simulink model "tppr2"  (R2020a)
settings: Solver=ode45  StartTime=0.0  StopTime=10  RelTol=1e-8
libraries: simulink x4
settings Model: Creator=dot  LastModifiedBy=dot

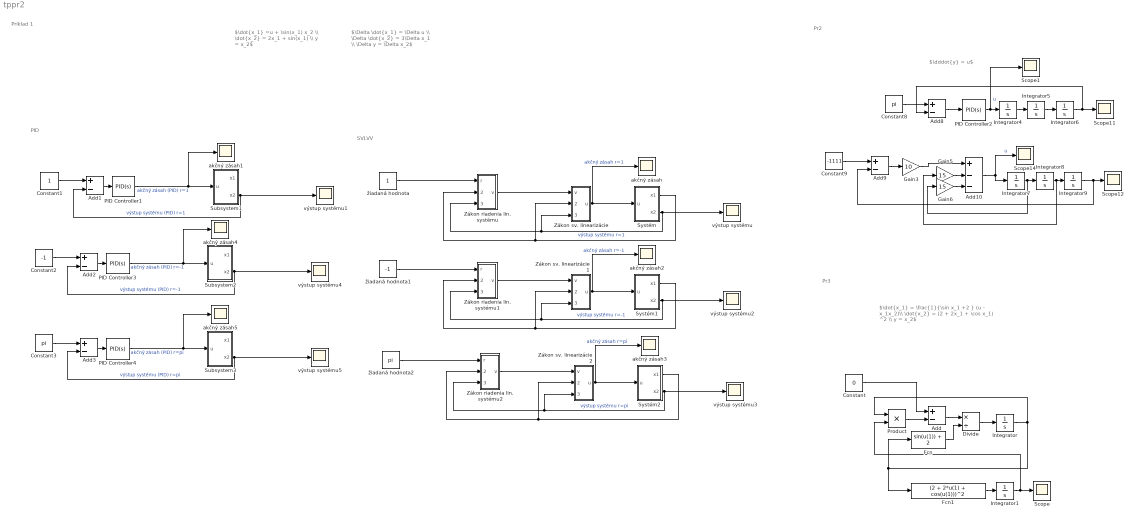
== system tppr2 ==
  note: Pr3
  note: Pr2
  note: Príklad 1
  note: SVLVV
  note: PID
  note: $\dot{x_1} =u + \sin(x_1) x_2 \\ \dot{x_2} = 2x_1 + sin(x_1) \\ y = x_2$
  note: $\dddot{y} = u$
  note: $\dot{x_1} = \frac{1}{\sin x_1 +2 } (u - x_1x_2)\\ \dot{x_2} = (2 + 2x_1 + \cos x_1) ^2 \\ y = x_2$
  note: $\Delta \dot{x_1} = \Delta u \\ \Delta \dot{x_2} = 3\Delta x_1 \\ \Delta y = \Delta x_2$
  Add{,1..3,8..9} (6 alike) : Sum  Inputs=+-
  Add10 : Sum  Inputs=+--
  Constant : Constant  Value=0
  Constant1 : Constant
  Constant2 : Constant  Value=-1
  Constant3 : Constant  Value=pi
  Constant8 : Constant  Value=pi
  Constant9 : Constant  Value=-1111
  Divide : Product  Inputs=*/
  Fcn : Fcn  Expr=sin(u(1)) + 2
  Fcn1 : Fcn  Expr=(2 + 2*u(1) + cos(u(1)))^2
  Gain3 : Gain  Gain=10
  Gain5 : Gain  Gain=15
  Gain6 : Gain  Gain=15
  Integrator : Integrator  InitialCondition=-1.18715
  Integrator1 : Integrator
  Integrator{4..9} (6 alike) : Integrator  InitialCondition=pi/2
  PID Controller1 : simulink/Continuous/PID Controller  Controller=PID  Form=Parallel  TimeDomain=Continuous-time  UseExternalTs=off  SampleTime=-1  IntegratorMethod=Forward Euler  FilterMethod=Forward Euler  ControllerParametersSource=internal  P=2/3  I=1.25/3  D=0.25/3  UseFilter=on  N=114.28279760416  TunerSelectOption=Transfer Function Based (PID Tuner App)  InitialConditionSource=internal  InitialConditionForIntegrator=0  InitialConditionForFilter=0  DifferentiatorICPrevScaledInput=0  ExternalReset=none  TrackingMode=off  Kt=1  LimitOutput=off  UpperSaturationLimit=inf  LowerSaturationLimit=-inf  LinearizeAsGain=on  AntiWindupMode=none  Kb=1  POutMin=[]  POutMax=[]  IOutMin=[]  IOutMax=[]  DOutMin=[]  DOutMax=[]  NOutMin=[]  NOutMax=[]  SumOutMin=[]  SumOutMax=[]  SaturationOutMin=[]  SaturationOutMax=[]  PParamMin=[]  PParamMax=[]  IParamMin=[]  IParamMax=[]  DParamMin=[]  DParamMax=[]  NParamMin=[]  NParamMax=[]  KbParamMin=[]  KbParamMax=[]  KtParamMin=[]  KtParamMax=[]  KbOutMin=[]  KbOutMax=[]  KtOutMin=[]  KtOutMax=[]  IntegratorOutMin=[]  IntegratorOutMax=[]  FilterOutMin=[]  FilterOutMax=[]  SumI1OutMin=[]  SumI1OutMax=[]  SumI2OutMin=[]  SumI2OutMax=[]  SumI3OutMin=[]  SumI3OutMax=[]  SumI4OutMin=[]  SumI4OutMax=[]  SumDOutMin=[]  SumDOutMax=[]  DifferentiatorOutMin=[]  DifferentiatorOutMax=[]  FilterDiffOutCoefMin=[]  FilterDiffOutCoefMax=[]  ReciprocalOutMin=[]  ReciprocalOutMax=[]  SumDenOutMin=[]  SumDenOutMax=[]  SumNumOutMin=[]  SumNumOutMax=[]  DivideOutMin=[]  DivideOutMax=[]  UdiffTsProdOutMin=[]  UdiffTsProdOutMax=[]  NTsProdOutMin=[]  NTsProdOutMax=[]  UintegralTsProdOutMin=[]  UintegralTsProdOutMax=[]  UngainTsProdOutMin=[]  UngainTsProdOutMax=[]  IntegratorContinuousStateAttributes=''  IntegratorStateMustResolveToSignalObject=off  IntegratorRTWStateStorageClass=Auto  FilterContinuousStateAttributes=''  FilterStateMustResolveToSignalObject=off  FilterRTWStateStorageClass=Auto  ParallelPVariant=InternalParameters  IdealPVariant=Disabled  IVariant=InternalParameters  DVariant=InternalParameters  IntegratorVariant=Continuous  SatVariant=Disabled  AWVariant=Passthrough  PCopyVariant=Disabled  TRVariant=Disabled  FdbkBlocksVariant=Forward  IdealPFdbkVariant=Disabled  SatFdbkVariant=Disabled  DerivativeFilterVariant=ContFilter  NVariant=InternalParameters  NCopyVariant=Disabled  FilterICVariant=InternalICsFilter  IntegratorICVariant=InternalICs  ExternalResetVariant=Disabled  TRSumVariant=Passthrough  SumFdbkVariant=Disabled  SumVariant=Sum_PID  TsampFilterVariant=InternalTs  TsampNgainVariant=Passthrough  TsampIntegralVariant=Passthrough
  PID Controller2 : simulink/Continuous/PID Controller  Controller=PID  Form=Parallel  TimeDomain=Continuous-time  UseExternalTs=off  SampleTime=-1  IntegratorMethod=Forward Euler  FilterMethod=Forward Euler  ControllerParametersSource=internal  P=20.1650988848254  I=19.5294021366559  D=3.60985208452342  UseFilter=on  N=386.119892426795  TunerSelectOption=Transfer Function Based (PID Tuner App)  InitialConditionSource=internal  InitialConditionForIntegrator=0  InitialConditionForFilter=0  DifferentiatorICPrevScaledInput=0  ExternalReset=none  TrackingMode=off  Kt=1  LimitOutput=off  UpperSaturationLimit=inf  LowerSaturationLimit=-inf  LinearizeAsGain=on  AntiWindupMode=none  Kb=1  POutMin=[]  POutMax=[]  IOutMin=[]  IOutMax=[]  DOutMin=[]  DOutMax=[]  NOutMin=[]  NOutMax=[]  SumOutMin=[]  SumOutMax=[]  SaturationOutMin=[]  SaturationOutMax=[]  PParamMin=[]  PParamMax=[]  IParamMin=[]  IParamMax=[]  DParamMin=[]  DParamMax=[]  NParamMin=[]  NParamMax=[]  KbParamMin=[]  KbParamMax=[]  KtParamMin=[]  KtParamMax=[]  KbOutMin=[]  KbOutMax=[]  KtOutMin=[]  KtOutMax=[]  IntegratorOutMin=[]  IntegratorOutMax=[]  FilterOutMin=[]  FilterOutMax=[]  SumI1OutMin=[]  SumI1OutMax=[]  SumI2OutMin=[]  SumI2OutMax=[]  SumI3OutMin=[]  SumI3OutMax=[]  SumI4OutMin=[]  SumI4OutMax=[]  SumDOutMin=[]  SumDOutMax=[]  DifferentiatorOutMin=[]  DifferentiatorOutMax=[]  FilterDiffOutCoefMin=[]  FilterDiffOutCoefMax=[]  ReciprocalOutMin=[]  ReciprocalOutMax=[]  SumDenOutMin=[]  SumDenOutMax=[]  SumNumOutMin=[]  SumNumOutMax=[]  DivideOutMin=[]  DivideOutMax=[]  UdiffTsProdOutMin=[]  UdiffTsProdOutMax=[]  NTsProdOutMin=[]  NTsProdOutMax=[]  UintegralTsProdOutMin=[]  UintegralTsProdOutMax=[]  UngainTsProdOutMin=[]  UngainTsProdOutMax=[]  IntegratorContinuousStateAttributes=''  IntegratorStateMustResolveToSignalObject=off  IntegratorRTWStateStorageClass=Auto  FilterContinuousStateAttributes=''  FilterStateMustResolveToSignalObject=off  FilterRTWStateStorageClass=Auto  ParallelPVariant=InternalParameters  IdealPVariant=Disabled  IVariant=InternalParameters  DVariant=InternalParameters  IntegratorVariant=Continuous  SatVariant=Disabled  AWVariant=Passthrough  PCopyVariant=Disabled  TRVariant=Disabled  FdbkBlocksVariant=Forward  IdealPFdbkVariant=Disabled  SatFdbkVariant=Disabled  DerivativeFilterVariant=ContFilter  NVariant=InternalParameters  NCopyVariant=Disabled  FilterICVariant=InternalICsFilter  IntegratorICVariant=InternalICs  ExternalResetVariant=Disabled  TRSumVariant=Passthrough  SumFdbkVariant=Disabled  SumVariant=Sum_PID  TsampFilterVariant=InternalTs  TsampNgainVariant=Passthrough  TsampIntegralVariant=Passthrough
  PID Controller3 : simulink/Continuous/PID Controller  Controller=PID  Form=Parallel  TimeDomain=Continuous-time  UseExternalTs=off  SampleTime=-1  IntegratorMethod=Forward Euler  FilterMethod=Forward Euler  ControllerParametersSource=internal  P=2/3  I=1.25/3  D=0.25/3  UseFilter=on  N=114.28279760416  TunerSelectOption=Transfer Function Based (PID Tuner App)  InitialConditionSource=internal  InitialConditionForIntegrator=0  InitialConditionForFilter=0  DifferentiatorICPrevScaledInput=0  ExternalReset=none  TrackingMode=off  Kt=1  LimitOutput=off  UpperSaturationLimit=inf  LowerSaturationLimit=-inf  LinearizeAsGain=on  AntiWindupMode=none  Kb=1  POutMin=[]  POutMax=[]  IOutMin=[]  IOutMax=[]  DOutMin=[]  DOutMax=[]  NOutMin=[]  NOutMax=[]  SumOutMin=[]  SumOutMax=[]  SaturationOutMin=[]  SaturationOutMax=[]  PParamMin=[]  PParamMax=[]  IParamMin=[]  IParamMax=[]  DParamMin=[]  DParamMax=[]  NParamMin=[]  NParamMax=[]  KbParamMin=[]  KbParamMax=[]  KtParamMin=[]  KtParamMax=[]  KbOutMin=[]  KbOutMax=[]  KtOutMin=[]  KtOutMax=[]  IntegratorOutMin=[]  IntegratorOutMax=[]  FilterOutMin=[]  FilterOutMax=[]  SumI1OutMin=[]  SumI1OutMax=[]  SumI2OutMin=[]  SumI2OutMax=[]  SumI3OutMin=[]  SumI3OutMax=[]  SumI4OutMin=[]  SumI4OutMax=[]  SumDOutMin=[]  SumDOutMax=[]  DifferentiatorOutMin=[]  DifferentiatorOutMax=[]  FilterDiffOutCoefMin=[]  FilterDiffOutCoefMax=[]  ReciprocalOutMin=[]  ReciprocalOutMax=[]  SumDenOutMin=[]  SumDenOutMax=[]  SumNumOutMin=[]  SumNumOutMax=[]  DivideOutMin=[]  DivideOutMax=[]  UdiffTsProdOutMin=[]  UdiffTsProdOutMax=[]  NTsProdOutMin=[]  NTsProdOutMax=[]  UintegralTsProdOutMin=[]  UintegralTsProdOutMax=[]  UngainTsProdOutMin=[]  UngainTsProdOutMax=[]  IntegratorContinuousStateAttributes=''  IntegratorStateMustResolveToSignalObject=off  IntegratorRTWStateStorageClass=Auto  FilterContinuousStateAttributes=''  FilterStateMustResolveToSignalObject=off  FilterRTWStateStorageClass=Auto  ParallelPVariant=InternalParameters  IdealPVariant=Disabled  IVariant=InternalParameters  DVariant=InternalParameters  IntegratorVariant=Continuous  SatVariant=Disabled  AWVariant=Passthrough  PCopyVariant=Disabled  TRVariant=Disabled  FdbkBlocksVariant=Forward  IdealPFdbkVariant=Disabled  SatFdbkVariant=Disabled  DerivativeFilterVariant=ContFilter  NVariant=InternalParameters  NCopyVariant=Disabled  FilterICVariant=InternalICsFilter  IntegratorICVariant=InternalICs  ExternalResetVariant=Disabled  TRSumVariant=Passthrough  SumFdbkVariant=Disabled  SumVariant=Sum_PID  TsampFilterVariant=InternalTs  TsampNgainVariant=Passthrough  TsampIntegralVariant=Passthrough
  PID Controller4 : simulink/Continuous/PID Controller  Controller=PID  Form=Parallel  TimeDomain=Continuous-time  UseExternalTs=off  SampleTime=-1  IntegratorMethod=Forward Euler  FilterMethod=Forward Euler  ControllerParametersSource=internal  P=2/3  I=1.25/3  D=0.25/3  UseFilter=on  N=114.28279760416  TunerSelectOption=Transfer Function Based (PID Tuner App)  InitialConditionSource=internal  InitialConditionForIntegrator=0  InitialConditionForFilter=0  DifferentiatorICPrevScaledInput=0  ExternalReset=none  TrackingMode=off  Kt=1  LimitOutput=off  UpperSaturationLimit=inf  LowerSaturationLimit=-inf  LinearizeAsGain=on  AntiWindupMode=none  Kb=1  POutMin=[]  POutMax=[]  IOutMin=[]  IOutMax=[]  DOutMin=[]  DOutMax=[]  NOutMin=[]  NOutMax=[]  SumOutMin=[]  SumOutMax=[]  SaturationOutMin=[]  SaturationOutMax=[]  PParamMin=[]  PParamMax=[]  IParamMin=[]  IParamMax=[]  DParamMin=[]  DParamMax=[]  NParamMin=[]  NParamMax=[]  KbParamMin=[]  KbParamMax=[]  KtParamMin=[]  KtParamMax=[]  KbOutMin=[]  KbOutMax=[]  KtOutMin=[]  KtOutMax=[]  IntegratorOutMin=[]  IntegratorOutMax=[]  FilterOutMin=[]  FilterOutMax=[]  SumI1OutMin=[]  SumI1OutMax=[]  SumI2OutMin=[]  SumI2OutMax=[]  SumI3OutMin=[]  SumI3OutMax=[]  SumI4OutMin=[]  SumI4OutMax=[]  SumDOutMin=[]  SumDOutMax=[]  DifferentiatorOutMin=[]  DifferentiatorOutMax=[]  FilterDiffOutCoefMin=[]  FilterDiffOutCoefMax=[]  ReciprocalOutMin=[]  ReciprocalOutMax=[]  SumDenOutMin=[]  SumDenOutMax=[]  SumNumOutMin=[]  SumNumOutMax=[]  DivideOutMin=[]  DivideOutMax=[]  UdiffTsProdOutMin=[]  UdiffTsProdOutMax=[]  NTsProdOutMin=[]  NTsProdOutMax=[]  UintegralTsProdOutMin=[]  UintegralTsProdOutMax=[]  UngainTsProdOutMin=[]  UngainTsProdOutMax=[]  IntegratorContinuousStateAttributes=''  IntegratorStateMustResolveToSignalObject=off  IntegratorRTWStateStorageClass=Auto  FilterContinuousStateAttributes=''  FilterStateMustResolveToSignalObject=off  FilterRTWStateStorageClass=Auto  ParallelPVariant=InternalParameters  IdealPVariant=Disabled  IVariant=InternalParameters  DVariant=InternalParameters  IntegratorVariant=Continuous  SatVariant=Disabled  AWVariant=Passthrough  PCopyVariant=Disabled  TRVariant=Disabled  FdbkBlocksVariant=Forward  IdealPFdbkVariant=Disabled  SatFdbkVariant=Disabled  DerivativeFilterVariant=ContFilter  NVariant=InternalParameters  NCopyVariant=Disabled  FilterICVariant=InternalICsFilter  IntegratorICVariant=InternalICs  ExternalResetVariant=Disabled  TRSumVariant=Passthrough  SumFdbkVariant=Disabled  SumVariant=Sum_PID  TsampFilterVariant=InternalTs  TsampNgainVariant=Passthrough  TsampIntegralVariant=Passthrough
  Product : Product
  Scope{,1,11..12,14} (5 alike) : Scope
  Subsystem1 : Subsystem
  Subsystem2 : Subsystem
  Subsystem3 : Subsystem
  Systém : Subsystem
  Systém1 : Subsystem
  Systém2 : Subsystem
  Zákon riadenia lin. systému : Subsystem
  Zákon riadenia lin. systému1 : Subsystem
  Zákon riadenia lin. systému2 : Subsystem
  Zákon sv. linearizácie : Subsystem
  Zákon sv. linearizácie1 : Subsystem
  Zákon sv. linearizácie2 : Subsystem
  akčný zásah{,1..5} (6 alike) : Scope
  výstup systému{,1..5} (6 alike) : Scope
  žiadaná hodnota : Constant
  žiadaná hodnota1 : Constant  Value=-1
  žiadaná hodnota2 : Constant  Value=pi
  wires:
  Integrator4/1 -> Integrator5/1
  Integrator5/1 -> Integrator6/1
  Constant8/1 -> Add8/1
  Integrator6/1 -> Add8/2, Scope11/1
  Add8/1 -> PID Controller2/1
  PID Controller2/1 -> Scope1/1, Integrator4/1  "u"
  Add10/1 -> Scope14/1, Integrator7/1  "u"
  Integrator9/1 -> Scope12/1, Add9/2
  Constant9/1 -> Add9/1
  Integrator8/1 -> Gain5/1, Integrator9/1
  Integrator7/1 -> Gain6/1, Integrator8/1
  Add9/1 -> Gain3/1
  Gain3/1 -> Add10/1
  Gain5/1 -> Add10/2
  Gain6/1 -> Add10/3
  Zákon sv. linearizácie/1(u) -> akčný zásah/1, Systém/1(u)  "akčný zásah r=1"
  Systém/1(x1) -> Zákon sv. linearizácie/2(x1), Zákon riadenia lin. systému/2(x1)
  Systém/2(x2) -> výstup systému/1, Zákon sv. linearizácie/3(x2), Zákon riadenia lin. systému/3(x2)  "výstup systému r=1"
  Zákon riadenia lin. systému/1(v) -> Zákon sv. linearizácie/1(v)
  žiadaná hodnota/1 -> Zákon riadenia lin. systému/1(r)
  Product/1 -> Add/2
  Add/1 -> Divide/1
  Divide/1 -> Integrator/1
  Integrator/1 -> Fcn1/1, Fcn/1, Product/1
  Constant/1 -> Add/1
  Fcn/1 -> Divide/2
  Integrator1/1 -> Scope/1, Product/2
  Fcn1/1 -> Integrator1/1
  Constant1/1 -> Add1/1
  PID Controller1/1 -> Subsystem1/1(u), akčný zásah1/1  "akčný zásah (PID) r=1"
  Subsystem1/2(x2) -> výstup systému1/1, Add1/2  "výstup systému (PID) r=1"
  Add1/1 -> PID Controller1/1
  žiadaná hodnota1/1 -> Zákon riadenia lin. systému1/1(r)
  Zákon riadenia lin. systému1/1(v) -> Zákon sv. linearizácie1/1(v)
  Systém1/2(x2) -> Zákon riadenia lin. systému1/3(x2), Zákon sv. linearizácie1/3(x2), výstup systému2/1  "výstup systému r=-1"
  Systém1/1(x1) -> Zákon riadenia lin. systému1/2(x1), Zákon sv. linearizácie1/2(x1)
  Zákon sv. linearizácie1/1(u) -> Systém1/1(u), akčný zásah2/1  "akčný zásah r=-1"
  Zákon sv. linearizácie2/1(u) -> akčný zásah3/1, Systém2/1(u)  "akčný zásah r=pi"
  Systém2/1(x1) -> Zákon sv. linearizácie2/2(x1), Zákon riadenia lin. systému2/2(x1)
  Systém2/2(x2) -> výstup systému3/1, Zákon sv. linearizácie2/3(x2), Zákon riadenia lin. systému2/3(x2)  "výstup systému r=pi"
  Zákon riadenia lin. systému2/1(v) -> Zákon sv. linearizácie2/1(v)
  žiadaná hodnota2/1 -> Zákon riadenia lin. systému2/1(r)
  Add2/1 -> PID Controller3/1
  Subsystem2/2(x2) -> Add2/2, výstup systému4/1  "výstup systému (PID) r=-1"
  PID Controller3/1 -> akčný zásah4/1, Subsystem2/1(u)  "akčný zásah (PID) r=-1"
  Constant2/1 -> Add2/1
  Constant3/1 -> Add3/1
  PID Controller4/1 -> Subsystem3/1(u), akčný zásah5/1  "akčný zásah (PID) r=pi"
  Subsystem3/2(x2) -> výstup systému5/1, Add3/2  "výstup systému (PID) r=pi"
  Add3/1 -> PID Controller4/1

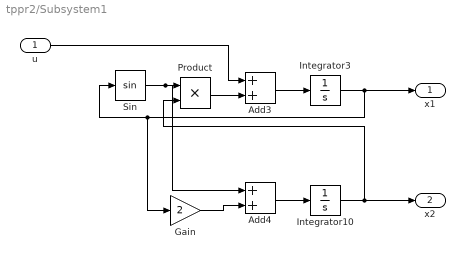
== system tppr2/Subsystem1 ==
  u : Inport
  Add3 : Sum
  Add4 : Sum
  Gain : Gain  Gain=2
  Integrator10 : Integrator
  Integrator3 : Integrator
  Product : Product
  Sin : Trigonometry
  x1 : Outport
  x2 : Outport  Port=2
  wires:
  Add4/1 -> Integrator10/1
  Gain/1 -> Add4/2
  u/1 -> Add3/1
  Add3/1 -> Integrator3/1
  Integrator3/1 -> Gain/1, Sin/1, x1/1
  Product/1 -> Add3/2
  Integrator10/1 -> Product/2, x2/1
  Sin/1 -> Add4/1, Product/1

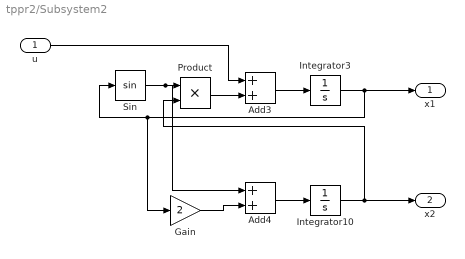
== system tppr2/Subsystem2 ==
  u : Inport
  Add3 : Sum
  Add4 : Sum
  Gain : Gain  Gain=2
  Integrator10 : Integrator
  Integrator3 : Integrator
  Product : Product
  Sin : Trigonometry
  x1 : Outport
  x2 : Outport  Port=2
  wires:
  Sin/1 -> Product/1, Add4/1
  Integrator10/1 -> x2/1, Product/2
  Product/1 -> Add3/2
  Integrator3/1 -> x1/1, Sin/1, Gain/1
  Add3/1 -> Integrator3/1
  u/1 -> Add3/1
  Gain/1 -> Add4/2
  Add4/1 -> Integrator10/1

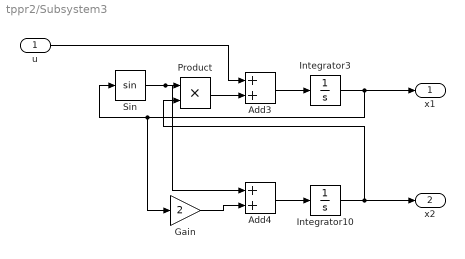
== system tppr2/Subsystem3 ==
  u : Inport
  Add3 : Sum
  Add4 : Sum
  Gain : Gain  Gain=2
  Integrator10 : Integrator
  Integrator3 : Integrator
  Product : Product
  Sin : Trigonometry
  x1 : Outport
  x2 : Outport  Port=2
  wires:
  Add4/1 -> Integrator10/1
  Gain/1 -> Add4/2
  u/1 -> Add3/1
  Add3/1 -> Integrator3/1
  Integrator3/1 -> Gain/1, Sin/1, x1/1
  Product/1 -> Add3/2
  Integrator10/1 -> Product/2, x2/1
  Sin/1 -> Add4/1, Product/1

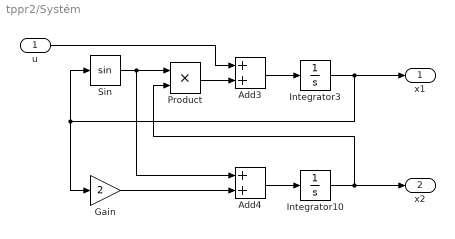
== system tppr2/Systém ==
  u : Inport
  Add3 : Sum
  Add4 : Sum
  Gain : Gain  Gain=2
  Integrator10 : Integrator
  Integrator3 : Integrator
  Product : Product
  Sin : Trigonometry
  x1 : Outport
  x2 : Outport  Port=2
  wires:
  Add4/1 -> Integrator10/1
  Gain/1 -> Add4/2
  u/1 -> Add3/1
  Add3/1 -> Integrator3/1
  Integrator3/1 -> Sin/1, Gain/1, x1/1
  Product/1 -> Add3/2
  Integrator10/1 -> Product/2, x2/1
  Sin/1 -> Product/1, Add4/1

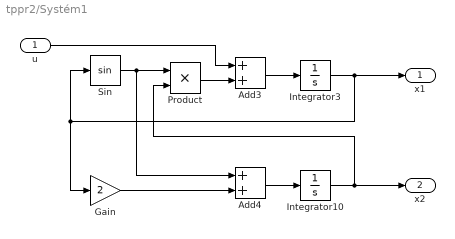
== system tppr2/Systém1 ==
  u : Inport
  Add3 : Sum
  Add4 : Sum
  Gain : Gain  Gain=2
  Integrator10 : Integrator
  Integrator3 : Integrator
  Product : Product
  Sin : Trigonometry
  x1 : Outport
  x2 : Outport  Port=2
  wires:
  Sin/1 -> Add4/1, Product/1
  Integrator10/1 -> x2/1, Product/2
  Product/1 -> Add3/2
  Integrator3/1 -> x1/1, Gain/1, Sin/1
  Add3/1 -> Integrator3/1
  u/1 -> Add3/1
  Gain/1 -> Add4/2
  Add4/1 -> Integrator10/1

== system tppr2/Systém2 ==
  u : Inport
  Add3 : Sum
  Add4 : Sum
  Gain : Gain  Gain=2
  Integrator10 : Integrator
  Integrator3 : Integrator
  Product : Product
  Sin : Trigonometry
  x1 : Outport
  x2 : Outport  Port=2
  wires:
  Add4/1 -> Integrator10/1
  Gain/1 -> Add4/2
  u/1 -> Add3/1
  Add3/1 -> Integrator3/1
  Integrator3/1 -> Sin/1, Gain/1, x1/1
  Product/1 -> Add3/2
  Integrator10/1 -> Product/2, x2/1
  Sin/1 -> Product/1, Add4/1

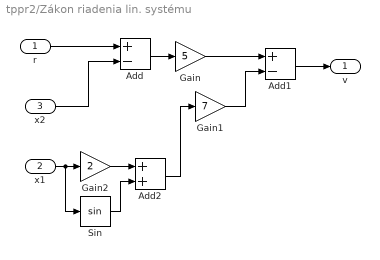
== system tppr2/Zákon riadenia lin. systému ==
  r : Inport
  x1 : Inport  Port=2
  x2 : Inport  Port=3
  Add : Sum  Inputs=+-
  Add1 : Sum  Inputs=+-
  Add2 : Sum
  Gain : Gain  Gain=5
  Gain1 : Gain  Gain=7
  Gain2 : Gain  Gain=2
  Sin : Trigonometry
  v : Outport
  wires:
  r/1 -> Add/1
  x1/1 -> Sin/1, Gain2/1
  Add/1 -> Gain/1
  Gain/1 -> Add1/1
  Add1/1 -> v/1
  Gain1/1 -> Add1/2
  Gain2/1 -> Add2/1
  Sin/1 -> Add2/2
  Add2/1 -> Gain1/1
  x2/1 -> Add/2

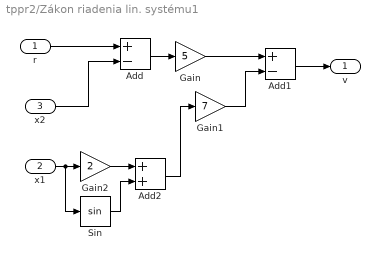
== system tppr2/Zákon riadenia lin. systému1 ==
  r : Inport
  x1 : Inport  Port=2
  x2 : Inport  Port=3
  Add : Sum  Inputs=+-
  Add1 : Sum  Inputs=+-
  Add2 : Sum
  Gain : Gain  Gain=5
  Gain1 : Gain  Gain=7
  Gain2 : Gain  Gain=2
  Sin : Trigonometry
  v : Outport
  wires:
  x2/1 -> Add/2
  Add2/1 -> Gain1/1
  Sin/1 -> Add2/2
  Gain2/1 -> Add2/1
  Gain1/1 -> Add1/2
  Add1/1 -> v/1
  Gain/1 -> Add1/1
  Add/1 -> Gain/1
  x1/1 -> Gain2/1, Sin/1
  r/1 -> Add/1

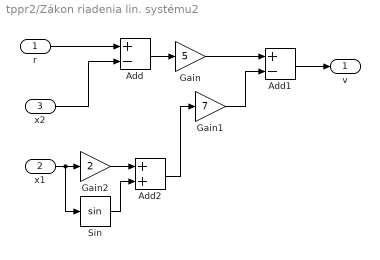
== system tppr2/Zákon riadenia lin. systému2 ==
  r : Inport
  x1 : Inport  Port=2
  x2 : Inport  Port=3
  Add : Sum  Inputs=+-
  Add1 : Sum  Inputs=+-
  Add2 : Sum
  Gain : Gain  Gain=5
  Gain1 : Gain  Gain=7
  Gain2 : Gain  Gain=2
  Sin : Trigonometry
  v : Outport
  wires:
  r/1 -> Add/1
  x1/1 -> Sin/1, Gain2/1
  Add/1 -> Gain/1
  Gain/1 -> Add1/1
  Add1/1 -> v/1
  Gain1/1 -> Add1/2
  Gain2/1 -> Add2/1
  Sin/1 -> Add2/2
  Add2/1 -> Gain1/1
  x2/1 -> Add/2

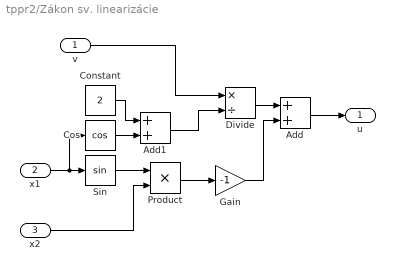
== system tppr2/Zákon sv. linearizácie ==
  v : Inport
  x1 : Inport  Port=2
  x2 : Inport  Port=3
  Add : Sum
  Add1 : Sum
  Constant : Constant  Value=2
  Cos : Trigonometry  Operator=cos
  Divide : Product  Inputs=*/
  Gain : Gain  Gain=-1
  Product : Product
  Sin : Trigonometry
  u : Outport
  wires:
  x1/1 -> Cos/1, Sin/1
  Sin/1 -> Product/1
  x2/1 -> Product/2
  Product/1 -> Gain/1
  Add/1 -> u/1
  Gain/1 -> Add/2
  Cos/1 -> Add1/2
  Constant/1 -> Add1/1
  Divide/1 -> Add/1
  v/1 -> Divide/1
  Add1/1 -> Divide/2

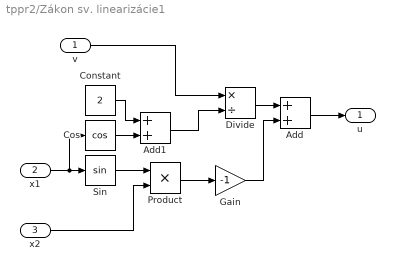
== system tppr2/Zákon sv. linearizácie1 ==
  v : Inport
  x1 : Inport  Port=2
  x2 : Inport  Port=3
  Add : Sum
  Add1 : Sum
  Constant : Constant  Value=2
  Cos : Trigonometry  Operator=cos
  Divide : Product  Inputs=*/
  Gain : Gain  Gain=-1
  Product : Product
  Sin : Trigonometry
  u : Outport
  wires:
  Add1/1 -> Divide/2
  v/1 -> Divide/1
  Divide/1 -> Add/1
  Constant/1 -> Add1/1
  Cos/1 -> Add1/2
  Gain/1 -> Add/2
  Add/1 -> u/1
  Product/1 -> Gain/1
  x2/1 -> Product/2
  Sin/1 -> Product/1
  x1/1 -> Sin/1, Cos/1

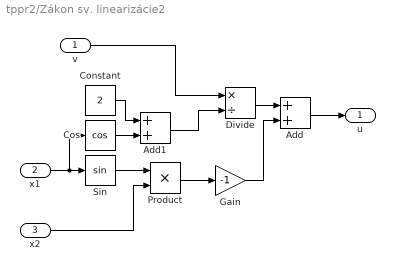
== system tppr2/Zákon sv. linearizácie2 ==
  v : Inport
  x1 : Inport  Port=2
  x2 : Inport  Port=3
  Add : Sum
  Add1 : Sum
  Constant : Constant  Value=2
  Cos : Trigonometry  Operator=cos
  Divide : Product  Inputs=*/
  Gain : Gain  Gain=-1
  Product : Product
  Sin : Trigonometry
  u : Outport
  wires:
  x1/1 -> Cos/1, Sin/1
  Sin/1 -> Product/1
  x2/1 -> Product/2
  Product/1 -> Gain/1
  Add/1 -> u/1
  Gain/1 -> Add/2
  Cos/1 -> Add1/2
  Constant/1 -> Add1/1
  Divide/1 -> Add/1
  v/1 -> Divide/1
  Add1/1 -> Divide/2
